simulink model "Control_system_v4"  (R2024b)
settings: Solver=FixedStepDiscrete  StartTime=0.0  StopTime=1000  FixedStep=1  RelTol=1e-3
undefined symbols (not defined in the file): A, B, C, Cj, D, Dj, I_a, K, L, start_time, Vk, Wk, x_eq, y_eq
settings Model: Creator=54238  LastModifiedBy=54238

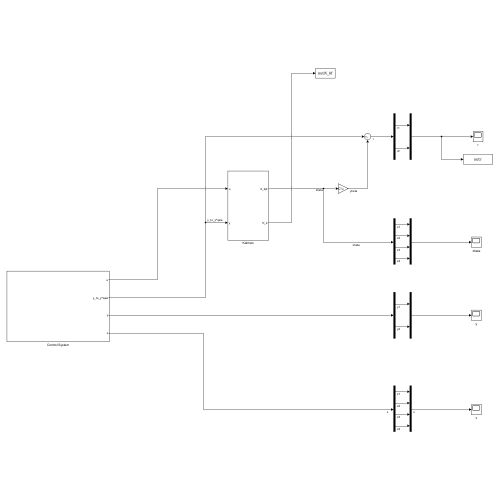
[thumbnail: Simulink's stored preview of the top-level diagram]
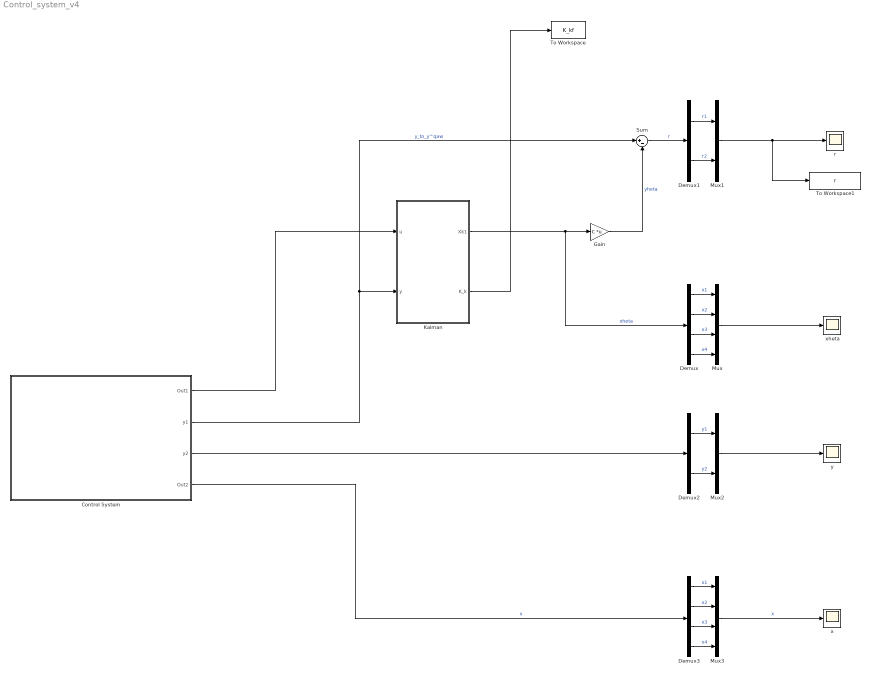
== system Control_system_v4 ==
  Control System : Subsystem
  Demux : Demux
  Demux1 : Demux  Outputs=2
  Demux2 : Demux  Outputs=2
  Demux3 : Demux
  Gain : Gain  Gain=C  Multiplication=Matrix(K*u)
  Kalman : Subsystem
  Mux : Mux
  Mux1 : Mux  Inputs=2
  Mux2 : Mux  Inputs=2
  Mux3 : Mux
  Sum : Sum  Inputs=|+-
  To Workspace : ToWorkspace  VariableName=K_kf  SampleTime=-1
  To Workspace1 : ToWorkspace  VariableName=r  SaveFormat=Timeseries  SampleTime=-1
  r : Scope
  x : Scope
  xheta : Scope
  y : Scope
  wires:
  Control System/1(Out1) -> Kalman/1(u)
  Gain/1 -> Sum/2  "yheta"
  Kalman/2(K_k) -> To Workspace/1
  Kalman/1(Xk1) -> Demux/1, Gain/1  "xheta"
  Mux/1 -> xheta/1
  Demux/4 -> Mux/4  "x4"
  Sum/1 -> Demux1/1  "r"
  Mux1/1 -> To Workspace1/1, r/1
  Demux/1 -> Mux/1  "x1"
  Demux/2 -> Mux/2  "x2"
  Demux/3 -> Mux/3  "x3"
  Demux1/1 -> Mux1/1  "r1"
  Demux1/2 -> Mux1/2  "r2"
  Demux2/1 -> Mux2/1  "y1"
  Control System/2(y1) -> Sum/1, Kalman/2(y)  "y_to_y^qaw"
  Mux2/1 -> y/1
  Demux2/2 -> Mux2/2  "y2"
  Control System/3(y2) -> Demux2/1
  Demux3/4 -> Mux3/4  "x4"
  Demux3/1 -> Mux3/1  "x1"
  Control System/4(Out2) -> Demux3/1  "x"
  Demux3/2 -> Mux3/2  "x2"
  Demux3/3 -> Mux3/3  "x3"
  Mux3/1 -> x/1  "x"

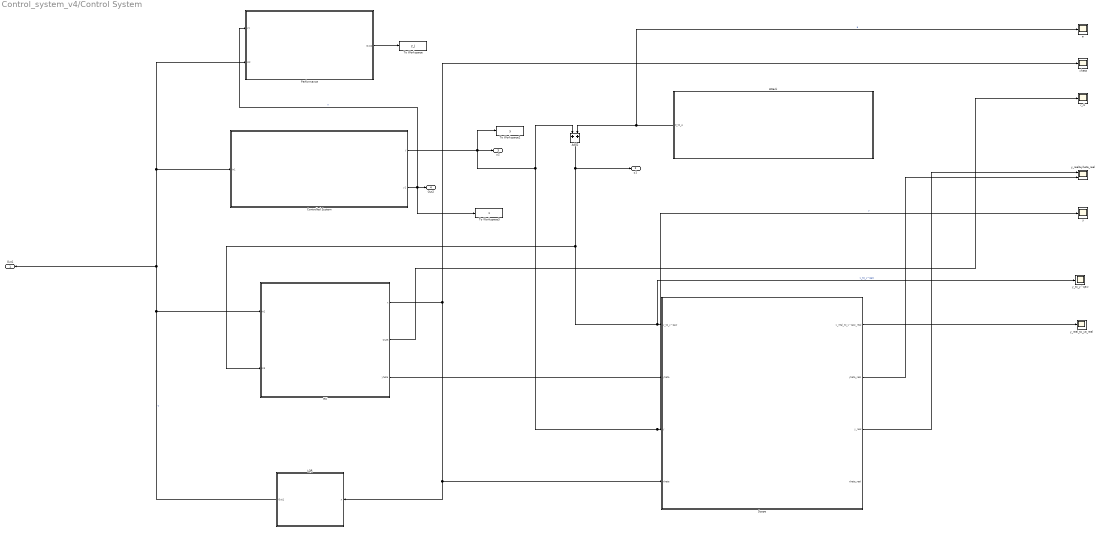
== system Control_system_v4/Control System ==
  Add2 : Sum
  Attack : Subsystem
  Controlled System : Subsystem
  LQR : Subsystem
  Performance : Subsystem
  RK : Subsystem
  Scope : Subsystem
  To Workspace : ToWorkspace  VariableName=y_j  SaveFormat=Timeseries  SampleTime=-1
  To Workspace2 : ToWorkspace  VariableName=y  SaveFormat=Timeseries  SampleTime=-1
  To Workspace3 : ToWorkspace  VariableName=x  SaveFormat=Timeseries  SampleTime=-1
  a : Scope
  r_rk : Scope
  xheta : Scope
  y : Scope
  y_real&yheta_real : Scope  NumInputPorts=2
  y_real_to_ya_real : Scope
  y_to_y^qaw : Scope
  Out1 : Outport  PortDimensions=[2,1]
  y1 : Outport  Port=2
  y2 : Outport  Port=3
  Out2 : Outport  Port=4
  wires:
  LQR/1(Out1) -> RK/1(In2), Performance/2(In2), Controlled System/1(In1), Out1/1  "u"
  RK/1(x) -> Scope/4(xheta), LQR/1(x), xheta/1
  RK/2(Out5) -> r_rk/1
  Controlled System/1(y) -> y/1, Scope/3(y), Add2/1, To Workspace2/1, y2/1  "y"
  Attack/1(0_to_a) -> a/1, Add2/2  "a"
  Add2/1 -> y_to_y^qaw/1, Scope/1(y_to_y^qaw), RK/2(In3), y1/1  "y_to_y^qaw"
  RK/3(yheta) -> Scope/2(yheta)
  Scope/3(y_real) -> y_real&yheta_real/1
  Scope/2(yheta_real) -> y_real&yheta_real/2
  Scope/1(y_real_to_y^qaw_real) -> y_real_to_ya_real/1
  Controlled System/2(y1) -> To Workspace3/1, Performance/1(y1), Out2/1  "x"
  Performance/1(Out2) -> To Workspace/1

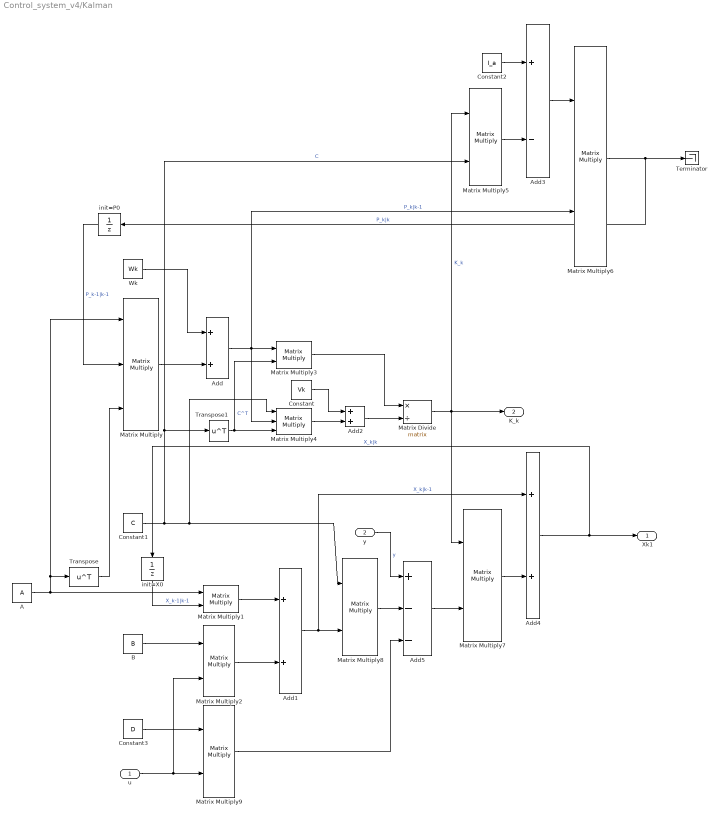
== system Control_system_v4/Kalman ==
  u : Inport  PortDimensions=[2,1]
  y : Inport  Port=2  PortDimensions=[2,1]
  A : Constant  Value=A
  Add{,1..2,4} (4 alike) : Sum
  Add3 : Sum  Inputs=+-
  Add5 : Sum  Inputs=+--
  B : Constant  Value=B
  Constant : Constant  Value=Vk
  Constant1 : Constant  Value=C
  Constant2 : Constant  Value=I_a
  Constant3 : Constant  Value=D
  Matrix Divide : Product  Inputs=*/  Multiplication=Matrix(*)
  Matrix Multiply : Product  Inputs=3  Multiplication=Matrix(*)
  Matrix Multiply{1..3,5..9} (8 alike) : Product  Multiplication=Matrix(*)
  Matrix Multiply4 : Product  Inputs=3  Multiplication=Matrix(*)
  Terminator : Terminator
  Transpose : Math  Operator=transpose  SignedPower=on  RndMeth=Zero
  Transpose1 : Math  Operator=transpose
  Wk : Constant  Value=Wk
  init=P0 : UnitDelay  SampleTime=-1  StateName=p0  HasFrameUpgradeWarning=on
  init=X0 : UnitDelay  InitialCondition=[5;5;2.044;1.399]  SampleTime=-1  HasFrameUpgradeWarning=on
  Xk1 : Outport  PortDimensions=[4,1]
  K_k : Outport  Port=2
  wires:
  Matrix Multiply2/1 -> Add1/2
  Add5/1 -> Matrix Multiply7/2
  Matrix Multiply6/1 -> Terminator/1, init=P0/1  "P_k|k"
  Constant1/1 -> Matrix Multiply4/1, Matrix Multiply8/1, Matrix Multiply5/2, Transpose1/1  "C"
  Add4/1 -> Xk1/1, init=X0/1  "X_k|k"
  Constant/1 -> Add2/1
  A/1 -> Matrix Multiply/1, Transpose/1, Matrix Multiply1/1
  Add1/1 -> Matrix Multiply8/2, Add4/1  "X_k|k-1"
  Constant2/1 -> Add3/1
  Add/1 -> Matrix Multiply3/1, Matrix Multiply4/2, Matrix Multiply6/2  "P_k|k-1"
  Add3/1 -> Matrix Multiply6/1
  init=X0/1 -> Matrix Multiply1/2  "X_k-1|k-1"
  Transpose/1 -> Matrix Multiply/3
  Matrix Multiply7/1 -> Add4/2
  init=P0/1 -> Matrix Multiply/2  "P_k-1|k-1"
  Matrix Multiply/1 -> Add/2
  Transpose1/1 -> Matrix Multiply4/3, Matrix Multiply3/2  "C^T"
  Wk/1 -> Add/1
  y/1 -> Add5/1  "y"
  Matrix Multiply5/1 -> Add3/2
  Matrix Divide/1 -> Matrix Multiply5/1, K_k/1, Matrix Multiply7/1  "K_k"
  u/1 -> Matrix Multiply2/2, Matrix Multiply9/2
  Matrix Multiply1/1 -> Add1/1
  Add2/1 -> Matrix Divide/2
  Matrix Multiply4/1 -> Add2/2
  Constant3/1 -> Matrix Multiply9/1
  Matrix Multiply8/1 -> Add5/2
  B/1 -> Matrix Multiply2/1
  Matrix Multiply9/1 -> Add5/3
  Matrix Multiply3/1 -> Matrix Divide/1

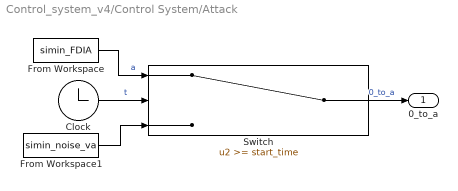
== system Control_system_v4/Control System/Attack ==
  Clock : Clock
  From Workspace : FromWorkspace  VariableName=simin_FDIA  SampleTime=-1
  From Workspace1 : FromWorkspace  VariableName=simin_noise_va  SampleTime=-1
  Switch : Switch  Threshold=start_time  SaturateOnIntegerOverflow=off  InputSameDT=off
  0_to_a : Outport
  wires:
  From Workspace1/1 -> Switch/3
  Clock/1 -> Switch/2  "t"
  From Workspace/1 -> Switch/1  "a"
  Switch/1 -> 0_to_a/1  "0_to_a"

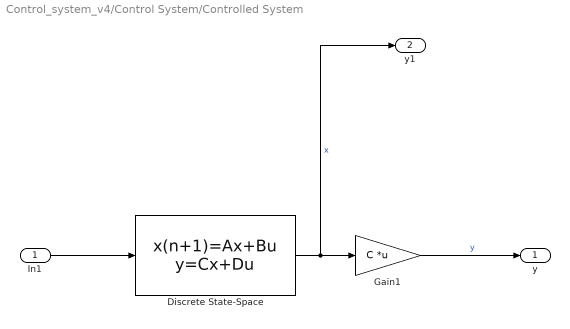
== system Control_system_v4/Control System/Controlled System ==
  In1 : Inport
  Discrete State-Space : DiscreteStateSpace  A=A  B=B  C=[1 0 0 0;0 1 0 0;0 0 1 0;0 0 0 1]  D=[0 0;0 0;0 0;0 0]  InitialCondition=[0 0 0 0]  SampleTime=-1
  Gain1 : Gain  Gain=C  Multiplication=Matrix(K*u)
  y : Outport
  y1 : Outport  Port=2
  wires:
  Gain1/1 -> y/1  "y"
  Discrete State-Space/1 -> y1/1, Gain1/1  "x"
  In1/1 -> Discrete State-Space/1

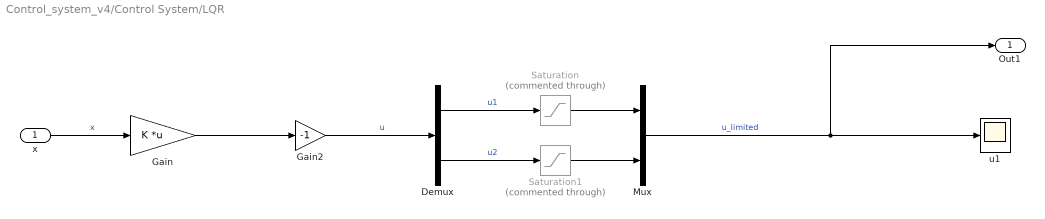
== system Control_system_v4/Control System/LQR ==
  x : Inport
  Demux : Demux  Outputs=2
  Gain : Gain  Gain=K  Multiplication=Matrix(K*u)
  Gain2 : Gain  Gain=-1
  Mux : Mux  Inputs=2
  Saturation : Saturate  Commented=through  UpperLimit=0.999  LowerLimit=-0.999
  Saturation1 : Saturate  Commented=through  UpperLimit=1.005  LowerLimit=-1.005
  u1 : Scope
  Out1 : Outport  PortDimensions=[2,1]
  wires:
  Saturation/1 -> Mux/1
  x/1 -> Gain/1  "x"
  Demux/1 -> Saturation/1  "u1"
  Mux/1 -> Out1/1, u1/1  "u_limited"
  Demux/2 -> Saturation1/1  "u2"
  Saturation1/1 -> Mux/2
  Gain/1 -> Gain2/1
  Gain2/1 -> Demux/1  "u"

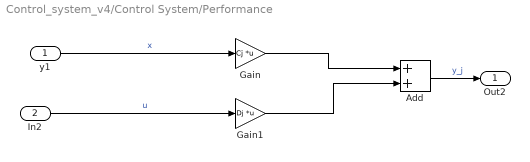
== system Control_system_v4/Control System/Performance ==
  y1 : Inport
  In2 : Inport  Port=2
  Add : Sum
  Gain : Gain  Gain=Cj  Multiplication=Matrix(K*u)
  Gain1 : Gain  Gain=Dj  Multiplication=Matrix(K*u)
  Out2 : Outport
  wires:
  In2/1 -> Gain1/1  "u"
  y1/1 -> Gain/1  "x"
  Gain/1 -> Add/1
  Add/1 -> Out2/1  "y_j"
  Gain1/1 -> Add/2

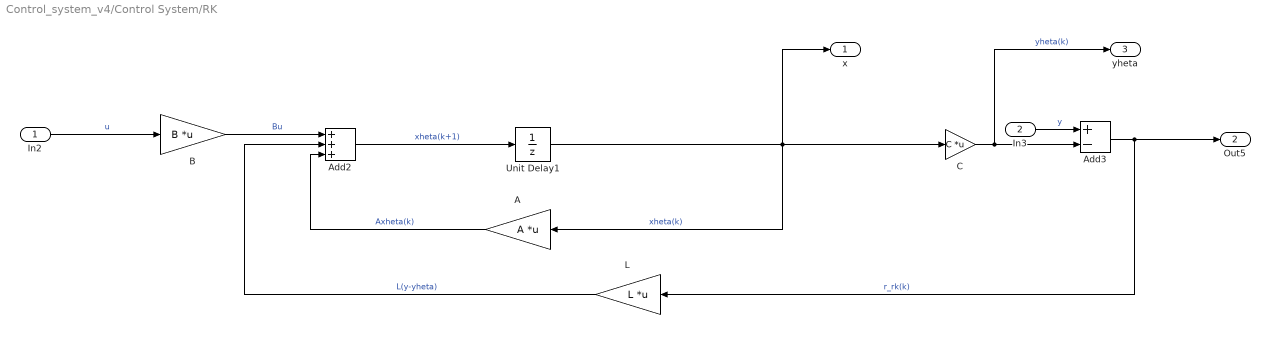
== system Control_system_v4/Control System/RK ==
  In2 : Inport
  In3 : Inport  Port=2
  A : Gain  Gain=A  Multiplication=Matrix(K*u)
  Add2 : Sum  Inputs=+++
  Add3 : Sum  Inputs=+-
  B : Gain  Gain=B  Multiplication=Matrix(K*u)
  C : Gain  Gain=C  Multiplication=Matrix(K*u)
  L : Gain  Gain=L  Multiplication=Matrix(K*u)
  Unit Delay1 : UnitDelay  SampleTime=-1  HasFrameUpgradeWarning=on
  x : Outport
  Out5 : Outport  Port=2
  yheta : Outport  Port=3
  wires:
  In3/1 -> Add3/1  "y"
  Add2/1 -> Unit Delay1/1  "xheta(k+1)"
  A/1 -> Add2/3  "Axheta(k)"
  B/1 -> Add2/1  "Bu"
  C/1 -> yheta/1, Add3/2  "yheta(k)"
  In2/1 -> B/1  "u"
  Unit Delay1/1 -> x/1, C/1, A/1  "xheta(k)"
  Add3/1 -> Out5/1, L/1  "r_rk(k)"
  L/1 -> Add2/2  "L(y-yheta)"

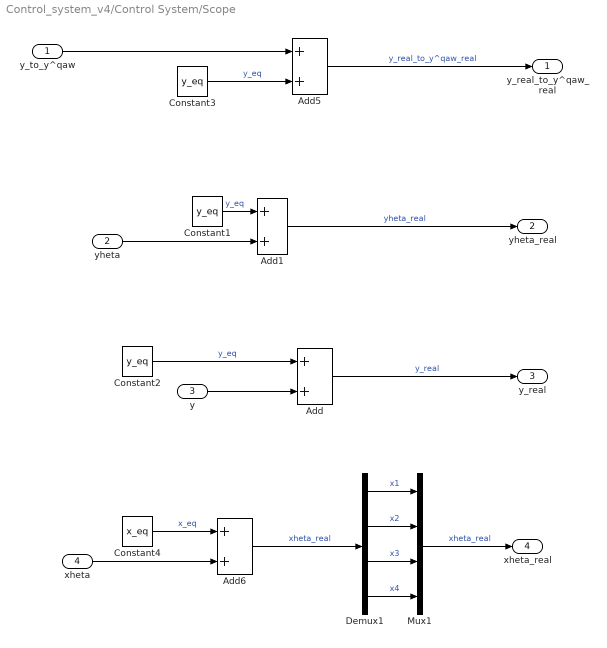
== system Control_system_v4/Control System/Scope ==
  y_to_y^qaw : Inport
  yheta : Inport  Port=2
  y : Inport  Port=3
  xheta : Inport  Port=4
  Add{,1,5..6} (4 alike) : Sum
  Constant1 : Constant  Value=y_eq  VectorParams1D=off
  Constant2 : Constant  Value=y_eq  VectorParams1D=off
  Constant3 : Constant  Value=y_eq  VectorParams1D=off
  Constant4 : Constant  Value=x_eq  VectorParams1D=off
  Demux1 : Demux
  Mux1 : Mux
  y_real_to_y^qaw_real : Outport
  yheta_real : Outport  Port=2
  y_real : Outport  Port=3
  xheta_real : Outport  Port=4
  wires:
  Demux1/1 -> Mux1/1  "x1"
  Constant4/1 -> Add6/1  "x_eq"
  Constant2/1 -> Add/1  "y_eq"
  Constant3/1 -> Add5/2  "y_eq"
  Add6/1 -> Demux1/1  "xheta_real"
  Add5/1 -> y_real_to_y^qaw_real/1  "y_real_to_y^qaw_real"
  Constant1/1 -> Add1/1  "y_eq"
  Demux1/3 -> Mux1/3  "x3"
  Demux1/2 -> Mux1/2  "x2"
  Demux1/4 -> Mux1/4  "x4"
  Add1/1 -> yheta_real/1  "yheta_real"
  yheta/1 -> Add1/2
  y/1 -> Add/2
  y_to_y^qaw/1 -> Add5/1
  Mux1/1 -> xheta_real/1  "xheta_real"
  Add/1 -> y_real/1  "y_real"
  xheta/1 -> Add6/2
